simulink model "gm_uz_pmsm_model_vnl"  (R2023b)
settings: Solver=FixedStepAuto  StartTime=0.0  StopTime=0.05  RelTol=1e-3
PreLoadFcn:
  | uz_pmsm_model_init_parameter
PostLoadFcn:
  | % Import the data from Excel for a lookup table
  | FluxMapData = readtable('C:\Users\Philipp\ultrazohm\ultrazohm_sw\ip_cores\uz_pmsm_model\FluxMapData_2023-05-26_13-07-57.csv');
  | % Row indices for lookup table
  | d_current_in_d_axis = FluxMapData(8:27,1:end);
  | % Column indices for lookup table
  | q_current_in_d_axis = FluxMapData(29:48,1:end);
  | % Output values for lookup table
  | d_Flux_d_axis = FluxMapData(50:69,1:end);
undefined symbols (not defined in the file or in its folder): ad1, ad2, ad3, ad4, ad5, ad6, aq1, aq2, aq3, aq4, aq5, aq6, d_current_d_Flux, d_current_q_Flux, entkopplung_dynamic, entkopplung_linear, entkopplung_static, Fid1_Giq1, Fid2_Giq2, Flux_d, Flux_q, friction_coefficient, inertia, Ki_Bo_d, Ki_Bo_q, Kp_Bo_d, Kp_Bo_q, L_d, L_q, Ldq, parameter_nachfuerung, polepair, praediktion_entkopplung_nonlinear, psi_pm, q_current_d_Flux, q_current_q_Flux, R_1, simulate_mechanical, simulate_nonlinear_modell, simulate_open_loop, static_friction_torque, tau_sum, ts, ts_regler
libraries: hdlmdlgenlib x16, slpidlib x6, simulink x4
(part 2 of 5)

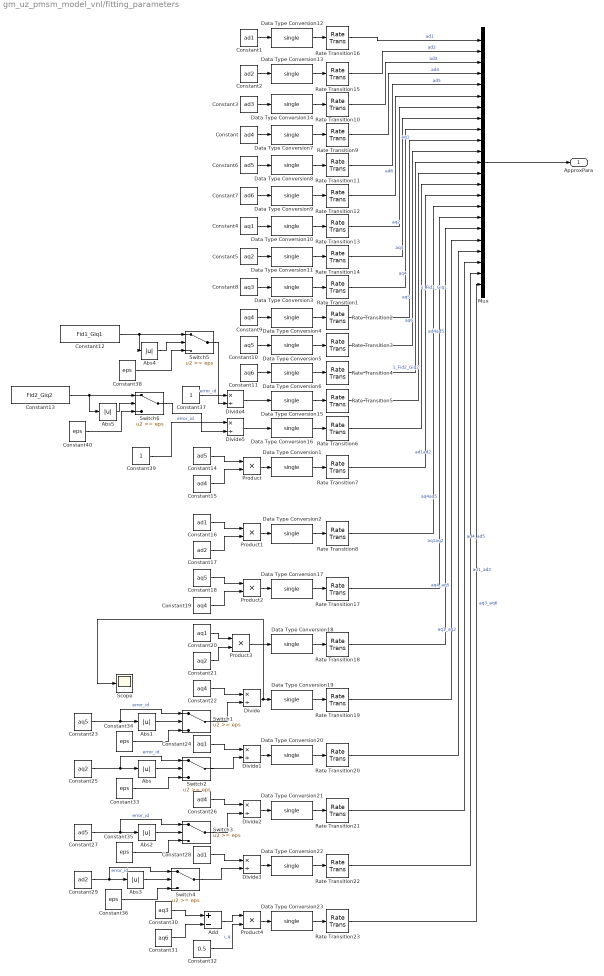
== system gm_uz_pmsm_model_vnl/fitting_parameters ==
  Abs{,1..5} (6 alike) : Abs  SaturateOnIntegerOverflow=off
  Add : Sum  Inputs=+-
  Constant : Constant  Value=ad4
  Constant1 : Constant  Value=ad1
  Constant10 : Constant  Value=aq5
  Constant11 : Constant  Value=aq6
  Constant12 : Constant  Value=Fid1_Giq1
  Constant13 : Constant  Value=Fid2_Giq2
  Constant14 : Constant  Value=ad5
  Constant15 : Constant  Value=ad4
  Constant16 : Constant  Value=ad1
  Constant17 : Constant  Value=ad2
  Constant18 : Constant  Value=aq5
  Constant19 : Constant  Value=aq4
  Constant2 : Constant  Value=ad2
  Constant20 : Constant  Value=aq1
  Constant21 : Constant  Value=aq2
  Constant22 : Constant  Value=aq4
  Constant23 : Constant  Value=aq5
  Constant24 : Constant  Value=aq1
  Constant25 : Constant  Value=aq2
  Constant26 : Constant  Value=ad4
  Constant27 : Constant  Value=ad5
  Constant28 : Constant  Value=ad1
  Constant29 : Constant  Value=ad2
  Constant3 : Constant  Value=ad3
  Constant30 : Constant  Value=aq3
  Constant31 : Constant  Value=aq6
  Constant32 : Constant  Value=0.5  OutDataTypeStr=double  SampleTime=-1
  Constant{33..36,38,40} (6 alike) : Constant  Value=eps  SampleTime=ts_regler
  Constant37 : Constant
  Constant39 : Constant
  Constant4 : Constant  Value=aq1
  Constant5 : Constant  Value=aq2
  Constant6 : Constant  Value=ad5
  Constant7 : Constant  Value=ad6
  Constant8 : Constant  Value=aq3
  Constant9 : Constant  Value=aq4
  Data Type Conversion{1..23} (23 alike) : DataTypeConversion  OutDataTypeStr=single  SaturateOnIntegerOverflow=off  RndMeth=Floor
  Divide{,1..5} (6 alike) : Product  Inputs=*/
  Mux : Mux  Inputs=23
  Product{,1..4} (5 alike) : Product
  Rate Transition{1..23} (23 alike) : RateTransition  OutPortSampleTime=ts
  Scope : Scope
  Switch{1..6} (6 alike) : Switch  Threshold=eps  SaturateOnIntegerOverflow=off  InputSameDT=off
  ApproxPara : Outport
  wires:
  Constant1/1 -> Data Type Conversion12/1
  Constant/1 -> Data Type Conversion7/1
  Rate Transition10/1 -> Mux/3  "ad3"
  Rate Transition14/1 -> Mux/8  "aq2"
  Constant3/1 -> Data Type Conversion14/1
  Rate Transition12/1 -> Mux/6  "ad6"
  Rate Transition16/1 -> Mux/1  "ad1"
  Rate Transition13/1 -> Mux/7  "aq1"
  Constant5/1 -> Data Type Conversion11/1
  Constant7/1 -> Data Type Conversion9/1
  Rate Transition15/1 -> Mux/2  "ad2"
  Rate Transition9/1 -> Mux/4  "ad4"
  Constant6/1 -> Data Type Conversion8/1
  Constant4/1 -> Data Type Conversion10/1
  Rate Transition11/1 -> Mux/5  "ad5"
  Constant2/1 -> Data Type Conversion13/1
  Rate Transition1/1 -> Mux/9  "aq3"
  Constant8/1 -> Data Type Conversion3/1
  Rate Transition2/1 -> Mux/10  "aq4"
  Constant9/1 -> Data Type Conversion4/1
  Rate Transition3/1 -> Mux/11  "aq5"
  Constant10/1 -> Data Type Conversion5/1
  Rate Transition4/1 -> Mux/12  "aq6"
  Constant11/1 -> Data Type Conversion6/1
  Rate Transition5/1 -> Mux/13  "1_Fid1_Giq1"
  Rate Transition6/1 -> Mux/14  "1_Fid2_Giq2"
  Data Type Conversion11/1 -> Rate Transition14/1
  Data Type Conversion10/1 -> Rate Transition13/1
  Data Type Conversion9/1 -> Rate Transition12/1
  Data Type Conversion12/1 -> Rate Transition16/1
  Data Type Conversion13/1 -> Rate Transition15/1
  Data Type Conversion14/1 -> Rate Transition10/1
  Data Type Conversion7/1 -> Rate Transition9/1
  Data Type Conversion8/1 -> Rate Transition11/1
  Data Type Conversion3/1 -> Rate Transition1/1
  Data Type Conversion4/1 -> Rate Transition2/1
  Data Type Conversion5/1 -> Rate Transition3/1
  Data Type Conversion6/1 -> Rate Transition4/1
  Data Type Conversion15/1 -> Rate Transition5/1
  Data Type Conversion16/1 -> Rate Transition6/1
  Constant14/1 -> Product/1
  Constant15/1 -> Product/2
  Product/1 -> Data Type Conversion1/1
  Data Type Conversion1/1 -> Rate Transition7/1
  Rate Transition7/1 -> Mux/15  "ad4ad5"
  Rate Transition8/1 -> Mux/16  "ad1ad2"
  Constant16/1 -> Product1/1
  Constant17/1 -> Product1/2
  Data Type Conversion2/1 -> Rate Transition8/1
  Product1/1 -> Data Type Conversion2/1
  Constant18/1 -> Product2/1
  Constant19/1 -> Product2/2
  Data Type Conversion17/1 -> Rate Transition17/1
  Product2/1 -> Data Type Conversion17/1
  Rate Transition18/1 -> Mux/18  "aq1aq2"
  Product3/1 -> Data Type Conversion18/1
  Data Type Conversion18/1 -> Rate Transition18/1
  Constant21/1 -> Product3/2
  Constant20/1 -> Product3/1
  Rate Transition17/1 -> Mux/17  "aq4aq5"
  Divide/1 -> Scope/1, Data Type Conversion19/1
  Data Type Conversion19/1 -> Rate Transition19/1
  Constant22/1 -> Divide/1
  Rate Transition19/1 -> Mux/19  "aq4_aq5"
  Constant24/1 -> Divide1/1
  Rate Transition20/1 -> Mux/20  "aq1_aq2"
  Divide1/1 -> Data Type Conversion20/1
  Data Type Conversion20/1 -> Rate Transition20/1
  Data Type Conversion21/1 -> Rate Transition21/1
  Divide2/1 -> Data Type Conversion21/1
  Rate Transition21/1 -> Mux/21  "ad4_ad5"
  Constant26/1 -> Divide2/1
  Constant28/1 -> Divide3/1
  Rate Transition22/1 -> Mux/22  "ad1_ad2"
  Divide3/1 -> Data Type Conversion22/1
  Data Type Conversion22/1 -> Rate Transition22/1
  Data Type Conversion23/1 -> Rate Transition23/1
  Constant30/1 -> Add/1
  Constant31/1 -> Add/2
  Rate Transition23/1 -> Mux/23  "aq3_aq6"
  Product4/1 -> Data Type Conversion23/1
  Constant32/1 -> Product4/2  "i_q"
  Add/1 -> Product4/1
  Mux/1 -> ApproxPara/1
  Constant25/1 -> Switch2/1, Abs/1  "error_id"
  Switch2/1 -> Divide1/2
  Abs/1 -> Switch2/2
  Constant33/1 -> Switch2/3
  Constant23/1 -> Switch1/1, Abs1/1  "error_id"
  Switch1/1 -> Divide/2
  Abs1/1 -> Switch1/2
  Constant34/1 -> Switch1/3
  Constant27/1 -> Switch3/1, Abs2/1  "error_id"
  Switch3/1 -> Divide2/2
  Abs2/1 -> Switch3/2
  Constant35/1 -> Switch3/3
  Constant29/1 -> Switch4/1, Abs3/1  "error_id"
  Switch4/1 -> Divide3/2
  Abs3/1 -> Switch4/2
  Constant36/1 -> Switch4/3
  Abs4/1 -> Switch5/2
  Constant38/1 -> Switch5/3
  Divide4/1 -> Data Type Conversion15/1
  Switch5/1 -> Divide4/2
  Constant12/1 -> Abs4/1, Switch5/1
  Constant37/1 -> Divide4/1  "error_id"
  Constant39/1 -> Divide5/1  "error_id"
  Constant13/1 -> Abs5/1, Switch6/1
  Constant40/1 -> Switch6/3
  Abs5/1 -> Switch6/2
  Divide5/1 -> Data Type Conversion16/1
  Switch6/1 -> Divide5/2

== system gm_uz_pmsm_model_vnl/model_parameters1 ==
  Bus Creator : BusCreator  Inputs=8
  Constant : Constant  Value=L_d
  Constant6 : Constant  Value=L_q
  Constant7 : Constant  Value=R_1
  Constant8 : Constant  Value=polepair
  Constant9 : Constant  Value=psi_pm
  Data Type Conversion{7..14} (8 alike) : DataTypeConversion  OutDataTypeStr=single  SaturateOnIntegerOverflow=off  RndMeth=Floor
  J : Constant  Value=1/inertia
  M_R0 : Constant  Value=static_friction_torque
  Rate Transition{9..16} (8 alike) : RateTransition  OutPortSampleTime=ts
  mu : Constant  Value=friction_coefficient
  Out1 : Outport
  wires:
  Data Type Conversion12/1 -> Rate Transition16/1
  Data Type Conversion7/1 -> Rate Transition9/1
  Rate Transition10/1 -> Bus Creator/3  "M_R0"
  Rate Transition14/1 -> Bus Creator/8  "psi_pm"
  Data Type Conversion14/1 -> Rate Transition10/1
  Rate Transition12/1 -> Bus Creator/6  "R_1"
  Rate Transition16/1 -> Bus Creator/1  "1_J"
  Rate Transition13/1 -> Bus Creator/7  "polepair"
  Bus Creator/1 -> Out1/1
  Data Type Conversion11/1 -> Rate Transition14/1
  Constant8/1 -> Data Type Conversion10/1
  Data Type Conversion9/1 -> Rate Transition12/1
  Rate Transition15/1 -> Bus Creator/2  "mu"
  Constant6/1 -> Data Type Conversion8/1
  Rate Transition9/1 -> Bus Creator/4  "1_L_d"
  J/1 -> Data Type Conversion12/1
  Data Type Conversion8/1 -> Rate Transition11/1
  Data Type Conversion10/1 -> Rate Transition13/1
  mu/1 -> Data Type Conversion13/1
  M_R0/1 -> Data Type Conversion14/1
  Rate Transition11/1 -> Bus Creator/5  "1_L_q"
  Data Type Conversion13/1 -> Rate Transition15/1
  Constant7/1 -> Data Type Conversion9/1
  Constant9/1 -> Data Type Conversion11/1
  Constant/1 -> Data Type Conversion7/1

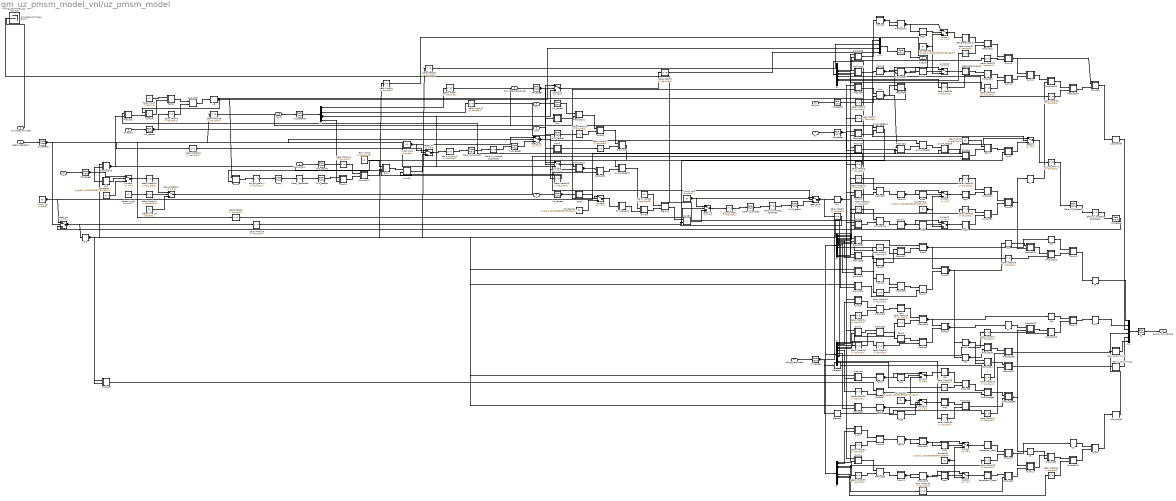
== system gm_uz_pmsm_model_vnl/uz_pmsm_model ==
  reset_integrators : Inport  OutDataTypeStr=boolean  PortDimensions=1  SampleTime=2e-06
  simulate_mechanical : Inport  Port=2  OutDataTypeStr=boolean  PortDimensions=1  SampleTime=2e-06
  simulate_nonlinear : Inport  Port=3  OutDataTypeStr=boolean  PortDimensions=1  SampleTime=2e-06
  reciprocal_J : Inport  Port=4  OutDataTypeStr=single  PortDimensions=1  SampleTime=2e-06
  mu : Inport  Port=5  OutDataTypeStr=single  PortDimensions=1  SampleTime=2e-06
  M_n0 : Inport  Port=6  OutDataTypeStr=single  PortDimensions=1  SampleTime=2e-06
  R1 : Inport  Port=7  OutDataTypeStr=single  PortDimensions=1  SampleTime=2e-06
  polepairs : Inport  Port=8  OutDataTypeStr=single  PortDimensions=1  SampleTime=2e-06
  Ld : Inport  Port=9  OutDataTypeStr=single  PortDimensions=1  SampleTime=2e-06
  Lq : Inport  Port=10  OutDataTypeStr=single  PortDimensions=1  SampleTime=2e-06
  psi_pm : Inport  Port=11  OutDataTypeStr=single  PortDimensions=1  SampleTime=2e-06
  fitting_parameter : Inport  Port=12  OutDataTypeStr=single  PortDimensions=[23]  SampleTime=2e-06
  inputs : Inport  Port=13  OutDataTypeStr=single  PortDimensions=[4]  SampleTime=2e-06
  Abs : Subsystem
      mask Display: disp('NFP\nabs');
  Constant{1..2,21..24} (6 alike) : Constant  Value=single(1.1920928955078125e-07)  OutDataTypeStr=single  SampleTime=1e-08
  Delay : RateTransition  OutPortSampleTimeOpt=Multiple of input port sample time  OutPortSampleTimeMultiple=200
  Delay1_lowered : RateTransition  OutPortSampleTimeOpt=Multiple of input port sample time  OutPortSampleTimeMultiple=200
  Delay1_lowered1 : RateTransition  OutPortSampleTimeOpt=Multiple of input port sample time  OutPortSampleTimeMultiple=200
  Delay1_lowered2 : RateTransition  OutPortSampleTimeOpt=Multiple of input port sample time  OutPortSampleTimeMultiple=200
  Delay1_lowered_absorbed : Delay  DelayLength=0
  Delay1_lowered_absorbed1 : Delay  DelayLength=0
  Delay1_lowered_absorbed2 : Delay  DelayLength=0
  Delay_absorbed : Delay  DelayLength=0
  Divide : Subsystem
      mask Display: disp('NFP\nmul');
  Divide1 : Subsystem
      mask Display: disp('NFP\nmul');
  Divide_recip : Subsystem
      mask Display: disp('NFP\nmath');
  Factor : Subsystem
      mask Display: disp('NFP\nmul');
  Factor_const : Constant  Value=single(1.5)  OutDataTypeStr=single  SampleTime=1e-08
  Gain : Subsystem
      mask Display: disp('NFP\nmul');
  Gain7 : Subsystem
      mask Display: disp('NFP\nmul');
  Gain71 : Subsystem
      mask Display: disp('NFP\nmul');
  Gain7_const : Constant  Value=single(2e-06)  OutDataTypeStr=single  SampleTime=1e-08
  Gain7_const1 : Constant  Value=single(2e-06)  OutDataTypeStr=single  SampleTime=1e-08
  Gain_const : Constant  Value=single(2e-06)  OutDataTypeStr=single  SampleTime=1e-08
  Gain_unaryminus : Subsystem
      mask Display: disp('NFP\numinus');
  Gain_unaryminus1 : Subsystem
      mask Display: disp('NFP\numinus');
  Initial_Val : Constant  Value=single(0)  OutDataTypeStr=single  SampleTime=1e-08
  Initial_Val1 : Constant  Value=single(0)  OutDataTypeStr=single  SampleTime=1e-08
  Initial_Val2 : Constant  Value=single(0)  OutDataTypeStr=single  SampleTime=1e-08
  Ldd_modell : hdlmdlgenlib/Buffer
  Log : Subsystem
      mask Display: disp('NFP\nmath');
  Log1 : Subsystem
      mask Display: disp('NFP\nmath');
  Log11 : Subsystem
      mask Display: disp('NFP\nmath');
  Log2 : Subsystem
      mask Display: disp('NFP\nmath');
  Lqq_modell : hdlmdlgenlib/Buffer
  Product : Subsystem
      mask Display: disp('NFP\nmul');
  Product1 : Subsystem
      mask Display: disp('NFP\nmul');
  Product10 : Subsystem
      mask Display: disp('NFP\nmul');
  Product101 : Subsystem
      mask Display: disp('NFP\nmul');
  Product102 : Subsystem
      mask Display: disp('NFP\nmul');
  Product103 : Subsystem
      mask Display: disp('NFP\nmul');
  Product104 : Subsystem
      mask Display: disp('NFP\nmul');
  Product11 : Subsystem
      mask Display: disp('NFP\nmul');
  Product110 : Subsystem
      mask Display: disp('NFP\nmul');
  Product111 : Subsystem
      mask Display: disp('NFP\nmul');
  Product12 : Subsystem
      mask Display: disp('NFP\nmul');
  Product121 : Subsystem
      mask Display: disp('NFP\nmul');
  Product13 : Subsystem
      mask Display: disp('NFP\nmul');
  Product131 : Subsystem
      mask Display: disp('NFP\nmul');
  Product14 : Subsystem
      mask Display: disp('NFP\nmul');
  Product141 : Subsystem
      mask Display: disp('NFP\nmul');
  Product15 : Subsystem
      mask Display: disp('NFP\nmul');
  Product151 : Subsystem
      mask Display: disp('NFP\nmul');
  Product16 : Subsystem
      mask Display: disp('NFP\nmul');
  Product17 : Subsystem
      mask Display: disp('NFP\nmul');
  Product18 : Subsystem
      mask Display: disp('NFP\nmul');
  Product19 : Subsystem
      mask Display: disp('NFP\nmul');
  Product2 : Subsystem
      mask Display: disp('NFP\nmul');
  Product20 : Subsystem
      mask Display: disp('NFP\nmul');
  Product201 : Subsystem
      mask Display: disp('NFP\nmul');
  Product202 : Subsystem
      mask Display: disp('NFP\nmul');
  Product203 : Subsystem
      mask Display: disp('NFP\nmul');
  Product204 : Subsystem
      mask Display: disp('NFP\nmul');
  Product205 : Subsystem
      mask Display: disp('NFP\nmul');
  Product206 : Subsystem
      mask Display: disp('NFP\nmul');
  Product207 : Subsystem
      mask Display: disp('NFP\nmul');
  Product21 : Subsystem
      mask Display: disp('NFP\nmul');
  Product22 : Subsystem
      mask Display: disp('NFP\nmul');
  Product23 : Subsystem
      mask Display: disp('NFP\nmul');
  Product24 : Subsystem
      mask Display: disp('NFP\nmul');
  Product25 : Subsystem
      mask Display: disp('NFP\nmul');
  Product3 : Subsystem
      mask Display: disp('NFP\nmul');
  Product31 : Subsystem
      mask Display: disp('NFP\nmul');
  Product32 : Subsystem
      mask Display: disp('NFP\nmul');
  Product33 : Subsystem
      mask Display: disp('NFP\nmul');
  Product34 : Subsystem
      mask Display: disp('NFP\nmul');
  Product35 : Subsystem
      mask Display: disp('NFP\nmul');
  Product4 : Subsystem
      mask Display: disp('NFP\nmul');
  Product41 : Subsystem
      mask Display: disp('NFP\nmul');
  Product42 : Subsystem
      mask Display: disp('NFP\nmul');
  Product43 : Subsystem
      mask Display: disp('NFP\nmul');
  Product5 : Subsystem
      mask Display: disp('NFP\nmul');
  Product51 : Subsystem
      mask Display: disp('NFP\nmul');
  Product52 : Subsystem
      mask Display: disp('NFP\nmul');
  Product6 : Subsystem
      mask Display: disp('NFP\nmul');
  Product61 : Subsystem
      mask Display: disp('NFP\nmul');
  Product7 : Subsystem
      mask Display: disp('NFP\nmul');
  Product71 : Subsystem
      mask Display: disp('NFP\nmul');
  Product8 : Subsystem
      mask Display: disp('NFP\nmul');
  Product9 : Subsystem
      mask Display: disp('NFP\nmul');
  Product91 : Subsystem
      mask Display: disp('NFP\nmul');
  Product92 : Subsystem
      mask Display: disp('NFP\nmul');
  Reciprocal1_recip : Subsystem
      mask Display: disp('NFP\nmath');
  Reciprocal1_recip1 : Subsystem
      mask Display: disp('NFP\nmath');
  Reciprocal_recip : Subsystem
      mask Display: disp('NFP\nmath');
  Reciprocal_recip1 : Subsystem
      mask Display: disp('NFP\nmath');
  Selector : Selector  IndexOptions=Index vector (dialog)  Indices=double(14)  OutputSizes=double(1)
  Selector1 : Selector  IndexOptions=Index vector (dialog)  Indices=double(13)  OutputSizes=double(1)
  Sign1 : Subsystem
      mask Display: disp('NFP\nsignum');
  Sum : Subsystem
      mask Display: disp('NFP\nadd');
  Sum1 : Subsystem
      mask Display: disp('NFP\nadd');
  Sum10 : Subsystem
      mask Display: disp('NFP\nadd');
  Sum101 : Subsystem
      mask Display: disp('NFP\nadd');
  Sum11 : Subsystem
      mask Display: disp('NFP\nadd');
  Sum12 : Subsystem
      mask Display: disp('NFP\nadd');
  Sum13 : Subsystem
      mask Display: disp('NFP\nadd');
  Sum14 : Subsystem
      mask Display: disp('NFP\nadd');
  Sum2 : Subsystem
      mask Display: disp('NFP\nadd');
  Sum21 : Subsystem
      mask Display: disp('NFP\nadd');
  Sum22 : Subsystem
      mask Display: disp('NFP\nadd');
  Sum23 : Subsystem
      mask Display: disp('NFP\nadd');
  Sum24 : Subsystem
      mask Display: disp('NFP\nadd');
  Sum3 : Subsystem
      mask Display: disp('NFP\nadd');
  Sum31 : Subsystem
      mask Display: disp('NFP\nadd');
  Sum32 : Subsystem
      mask Display: disp('NFP\nadd');
  Sum33 : Subsystem
      mask Display: disp('NFP\nadd');
  Sum3_stage2 : Subsystem
      mask Display: disp('NFP\nadd');
  Sum3_stage21 : Subsystem
      mask Display: disp('NFP\nadd');
  Sum3_stage3 : Subsystem
      mask Display: disp('NFP\nadd');
  Sum3_stage31 : Subsystem
      mask Display: disp('NFP\nadd');
  Sum4 : Subsystem
      mask Display: disp('NFP\nadd');
  Sum41 : Subsystem
      mask Display: disp('NFP\nadd');
  Sum4_stage2 : Subsystem
      mask Display: disp('NFP\nadd');
  Sum4_stage3 : Subsystem
      mask Display: disp('NFP\nadd');
  Sum5 : Subsystem
      mask Display: disp('NFP\nadd');
  Sum51 : Subsystem
      mask Display: disp('NFP\nadd');
  Sum52 : Subsystem
      mask Display: disp('NFP\nadd');
  Sum53 : Subsystem
      mask Display: disp('NFP\nadd');
  Sum6 : Subsystem
      mask Display: disp('NFP\nadd');
  Sum7 : Subsystem
      mask Display: disp('NFP\nadd');
  Sum71 : Subsystem
      mask Display: disp('NFP\nadd');
  Sum8 : Subsystem
      mask Display: disp('NFP\nadd');
  Switch{,1..6,8,11..14} (12 alike) : Switch  Criteria=u2 ~= 0  Threshold=double(0)  OutDataTypeStr=single  SampleTime=1e-08  SaturateOnIntegerOverflow=off  InputSameDT=off
  Tanh : Subsystem
      mask Display: disp('NFP\ntrig');
  Tanh1 : Subsystem
      mask Display: disp('NFP\ntrig');
  Tanh11 : Subsystem
      mask Display: disp('NFP\ntrig');
  Tanh12 : Subsystem
      mask Display: disp('NFP\ntrig');
  Tanh13 : Subsystem
      mask Display: disp('NFP\ntrig');
  Tanh2 : Subsystem
      mask Display: disp('NFP\ntrig');
  Tanh21 : Subsystem
      mask Display: disp('NFP\ntrig');
  Tanh3 : Subsystem
      mask Display: disp('NFP\ntrig');
  Tanh31 : Subsystem
      mask Display: disp('NFP\ntrig');
  Tanh4 : Subsystem
      mask Display: disp('NFP\ntrig');
  Tanh41 : Subsystem
      mask Display: disp('NFP\ntrig');
  Tanh5 : Subsystem
      mask Display: disp('NFP\ntrig');
  abs : Subsystem
      mask Display: disp('NFP\nabs');
  abs1 : Subsystem
      mask Display: disp('NFP\nabs');
  abs2 : Subsystem
      mask Display: disp('NFP\nabs');
  abs3 : Subsystem
      mask Display: disp('NFP\nabs');
  abs4 : Subsystem
      mask Display: disp('NFP\nabs');
  abs5 : Subsystem
      mask Display: disp('NFP\nabs');
  abs6 : Subsystem
      mask Display: disp('NFP\nabs');
  abs7 : Subsystem
      mask Display: disp('NFP\nabs');
  abs8 : Subsystem
      mask Display: disp('NFP\nabs');
  abs9 : Subsystem
      mask Display: disp('NFP\nabs');
  crp_out_delay{,1..3} (4 alike) : Delay  DelayLength=double(1)  InitialCondition=0  SampleTime=1e-08
  default_value : Constant  Value=double(1)  OutDataTypeStr=single  SampleTime=1e-08
  delayMatch{,1..13,15..46} (46 alike) : Delay  DelayLength=double(1)  InitialCondition=0  SampleTime=1e-08
  delayMatch14 : Delay  DelayLength=double(30)  InitialCondition=0  SampleTime=1e-08
  fitting_parameter_13_term13 : Terminator
  i_q : hdlmdlgenlib/Buffer
  in0_repeat : RateTransition  Integrity=off  Deterministic=off  OutPortSampleTimeOpt=Multiple of input port sample time  OutPortSampleTimeMultiple=1/200
  in10_repeat : RateTransition  Integrity=off  Deterministic=off  OutPortSampleTimeOpt=Multiple of input port sample time  OutPortSampleTimeMultiple=1/200
  in11_repeat : RateTransition  Integrity=off  Deterministic=off  OutPortSampleTimeOpt=Multiple of input port sample time  OutPortSampleTimeMultiple=1/200
  in12_repeat : RateTransition  Integrity=off  Deterministic=off  OutPortSampleTimeOpt=Multiple of input port sample time  OutPortSampleTimeMultiple=1/200
  in13_repeat : RateTransition  Integrity=off  Deterministic=off  OutPortSampleTimeOpt=Multiple of input port sample time  OutPortSampleTimeMultiple=1/200
  in14_repeat : RateTransition  Integrity=off  Deterministic=off  OutPortSampleTimeOpt=Multiple of input port sample time  OutPortSampleTimeMultiple=1/200
  in15_repeat : RateTransition  Integrity=off  Deterministic=off  OutPortSampleTimeOpt=Multiple of input port sample time  OutPortSampleTimeMultiple=1/200
  in1_repeat : RateTransition  Integrity=off  Deterministic=off  OutPortSampleTimeOpt=Multiple of input port sample time  OutPortSampleTimeMultiple=1/200
  in2_repeat : RateTransition  Integrity=off  Deterministic=off  OutPortSampleTimeOpt=Multiple of input port sample time  OutPortSampleTimeMultiple=1/200
  in3_repeat : RateTransition  Integrity=off  Deterministic=off  OutPortSampleTimeOpt=Multiple of input port sample time  OutPortSampleTimeMultiple=1/200
  in4_repeat : RateTransition  Integrity=off  Deterministic=off  OutPortSampleTimeOpt=Multiple of input port sample time  OutPortSampleTimeMultiple=1/200
  in5_repeat : RateTransition  Integrity=off  Deterministic=off  OutPortSampleTimeOpt=Multiple of input port sample time  OutPortSampleTimeMultiple=1/200
  in6_repeat : RateTransition  Integrity=off  Deterministic=off  OutPortSampleTimeOpt=Multiple of input port sample time  OutPortSampleTimeMultiple=1/200
  in7_repeat : RateTransition  Integrity=off  Deterministic=off  OutPortSampleTimeOpt=Multiple of input port sample time  OutPortSampleTimeMultiple=1/200
  in8_repeat : RateTransition  Integrity=off  Deterministic=off  OutPortSampleTimeOpt=Multiple of input port sample time  OutPortSampleTimeMultiple=1/200
  in9_repeat : RateTransition  Integrity=off  Deterministic=off  OutPortSampleTimeOpt=Multiple of input port sample time  OutPortSampleTimeMultiple=1/200
  mux : Mux  Inputs=6
  mux1 : Mux
  reset_in : Switch  Criteria=u2 ~= 0  Threshold=double(0)  OutDataTypeStr=single  SampleTime=1e-08  SaturateOnIntegerOverflow=off  InputSameDT=off
  reset_in1 : Switch  Criteria=u2 ~= 0  Threshold=double(0)  OutDataTypeStr=single  SampleTime=1e-08  SaturateOnIntegerOverflow=off  InputSameDT=off
  reset_in2 : Switch  Criteria=u2 ~= 0  Threshold=double(0)  OutDataTypeStr=single  SampleTime=1e-08  SaturateOnIntegerOverflow=off  InputSameDT=off
  reset_out : Switch  Criteria=u2 ~= 0  Threshold=double(0)  OutDataTypeStr=single  SampleTime=1e-08  SaturateOnIntegerOverflow=off  InputSameDT=off
  reset_out1 : Switch  Criteria=u2 ~= 0  Threshold=double(0)  OutDataTypeStr=single  SampleTime=1e-08  SaturateOnIntegerOverflow=off  InputSameDT=off
  reset_out2 : Switch  Criteria=u2 ~= 0  Threshold=double(0)  OutDataTypeStr=single  SampleTime=1e-08  SaturateOnIntegerOverflow=off  InputSameDT=off
  select_signal : Constant  Value=double(1)  OutDataTypeStr=boolean  SampleTime=1e-08
  simulate_nonlinear_term2 : Terminator
  t : RateTransition  OutPortSampleTimeOpt=Multiple of input port sample time  OutPortSampleTimeMultiple=200
  t1 : RateTransition  OutPortSampleTimeOpt=Multiple of input port sample time  OutPortSampleTimeMultiple=200
  t{7..19} (13 alike) : hdlmdlgenlib/Buffer
  t{2..5} (4 alike) : Demux  Outputs=23
  t6 : Demux
  zero_protection : Switch  Criteria=u2 ~= 0  Threshold=double(0)  OutDataTypeStr=single  SampleTime=1e-08  SaturateOnIntegerOverflow=off  InputSameDT=off
  outputs : Outport  SampleTime=2e-06
  approx_flux_testing : Outport  Port=2  SampleTime=2e-06
  wires:
  default_value/1 -> zero_protection/3
  zero_protection/1 -> Divide1/2(In2)
  reset_out1/1 -> Switch5/1, Switch14/1, Sign1/1(In1), Abs/1(In1), delayMatch45/1
  Selector1/1 -> delayMatch43/1
  Selector/1 -> delayMatch42/1
  delayMatch46/1 -> reset_in1/2
  reset_out/1 -> delayMatch15/1, t13/1
  select_signal/1 -> delayMatch14/1
  Switch8/1 -> delayMatch13/1
  Switch14/1 -> delayMatch9/1
  delayMatch7/1 -> mux1/1
  delayMatch8/1 -> mux1/2
  delayMatch16/1 -> reset_in/2
  reset_out2/1 -> delayMatch1/1, t14/1
  delayMatch14/1 -> zero_protection/2
  Gain/1(Out1) -> Sum32/1(In1)
  Sum3_stage31/1(Out1) -> Divide/1(In1)
  Sum3_stage21/1(Out1) -> Sum3_stage31/1(In1)
  Divide_recip/1(Out1) -> Divide/2(In2)
  abs9/1(Out1) -> Switch6/2
  Sum53/1(Out1) -> reset_in2/3
  Product43/1(Out1) -> Sum3_stage21/2(In2)
  Product35/1(Out1) -> Sum33/1(In1)
  Sum33/1(Out1) -> Factor/2(In2)
  Sum8/1(Out1) -> crp_out_delay1/1
  Product42/1(Out1) -> Sum8/2(In2)
  Sum52/1(Out1) -> Product42/1(In1)
  Product121/1(Out1) -> Sum52/1(In1)
  Abs/1(Out1) -> Product121/2(In2)
  Sum32/1(Out1) -> reset_in1/3
  Product111/1(Out1) -> Gain/2(In2)
  Sum14/1(Out1) -> Product111/2(In2)
  Sign1/1(Out1) -> delayMatch11/1
  Product131/1(Out1) -> Product21/2(In2), Product34/1(In1)
  Product110/1(Out1) -> Product2/2(In2), Product34/2(In2)
  Product25/1(Out1) -> Tanh13/1(In1)
  Tanh13/1(Out1) -> Product151/1(In1), Product151/2(In2)
  Product151/1(Out1) -> Switch13/1, abs8/1(In1)
  abs8/1(Out1) -> Switch13/2
  Reciprocal1_recip1/1(Out1) -> Product33/1(In1)
  Sum41/1(Out1) -> Sum24/2(In2)
  Sum24/1(Out1) -> Product206/1(In1)
  Product206/1(Out1) -> Product207/1(In1)
  Sum13/1(Out1) -> Sum101/1(In1), Sum24/1(In1)
  Reciprocal_recip1/1(Out1) -> Product19/1(In1)
  abs7/1(Out1) -> Switch4/2
  Product141/1(Out1) -> Switch4/1, abs7/1(In1)
  Tanh31/1(Out1) -> Product141/1(In1), Product141/2(In2)
  Product18/1(Out1) -> Tanh31/1(In1)
  Sum4/1(Out1) -> Sum23/1(In1), t19/1
  Sum23/1(Out1) -> t12/1, t15/1
  Product204/1(Out1) -> Product205/1(In1)
  Product41/1(Out1) -> Sum51/1(In1)
  Tanh12/1(Out1) -> Product32/1(In1)
  Product24/1(Out1) -> Tanh12/1(In1)
  Sum12/1(Out1) -> Sum23/2(In2)
  Product61/1(Out1) -> Sum12/2(In2)
  Product52/1(Out1) -> Sum4/1(In1)
  Product17/1(Out1) -> Sum4/2(In2)
  Tanh5/1(Out1) -> Product17/1(In1)
  Product16/1(Out1) -> Tanh5/1(In1)
  Tanh41/1(Out1) -> Switch3/1, abs6/1(In1)
  abs6/1(Out1) -> Switch3/2
  abs5/1(Out1) -> Switch12/2
  Tanh21/1(Out1) -> Switch12/1, abs5/1(In1)
  Log11/1(Out1) -> Product91/2(In2)
  Product91/1(Out1) -> Sum51/2(In2)
  Log2/1(Out1) -> Product41/2(In2)
  Product202/1(Out1) -> Product203/1(In1)
  Sum22/1(Out1) -> t11/1, t17/1
  Product102/1(Out1) -> Product103/1(In1)
  Product13/1(Out1) -> Sum22/1(In1), t18/1
  Tanh/1(Out1) -> Product13/1(In1)
  Product11/1(Out1) -> Tanh/1(In1)
  Sum3/1(Out1) -> Product11/1(In1)
  Product4/1(Out1) -> Tanh2/1(In1)
  Tanh2/1(Out1) -> Switch2/1, abs4/1(In1)
  abs4/1(Out1) -> Switch2/2
  Log/1(Out1) -> Product6/1(In1)
  Product6/1(Out1) -> Sum3_stage2/1(In1)
  Sum3_stage2/1(Out1) -> Sum3_stage3/1(In1)
  Product12/1(Out1) -> Sum3_stage3/2(In2)
  Log1/1(Out1) -> Product12/1(In1)
  abs3/1(Out1) -> Switch11/2
  Product51/1(Out1) -> Tanh3/1(In1)
  Product7/1(Out1) -> Sum3_stage2/2(In2)
  Product8/1(Out1) -> Product7/1(In1)
  Product10/1(Out1) -> Product101/1(In1)
  Product1/1(Out1) -> Sum21/1(In1), t16/1
  Reciprocal1_recip/1(Out1) -> Product31/1(In1)
  abs2/1(Out1) -> Switch1/2
  Product15/1(Out1) -> Switch1/1, abs2/1(In1)
  Tanh11/1(Out1) -> Product15/1(In1), Product15/2(In2)
  Product23/1(Out1) -> Tanh11/1(In1)
  Sum11/1(Out1) -> Product23/1(In1)
  Product/1(Out1) -> Tanh4/1(In1)
  Sum2/1(Out1) -> Product/1(In1)
  Tanh4/1(Out1) -> Product14/1(In1), Product14/2(In2)
  Product14/1(Out1) -> Switch/1, abs1/1(In1)
  abs1/1(Out1) -> Switch/2
  Reciprocal_recip/1(Out1) -> Product1/1(In1)
  Tanh1/1(Out1) -> Product3/1(In1)
  Product22/1(Out1) -> Tanh1/1(In1)
  Sum1/1(Out1) -> Product22/1(In1)
  Product201/1(Out1) -> Gain_unaryminus1/1(In1)
  Product20/1(Out1) -> Product201/1(In1)
  Product9/1(Out1) -> Sum4_stage3/2(In2)
  Sum4_stage3/1(Out1) -> Divide1/1(In1)
  Sum4_stage2/1(Out1) -> Sum4_stage3/1(In1)
  Sum/1(Out1) -> Product35/1(In1), Product21/1(In1)
  Product5/1(Out1) -> Sum/1(In1)
  abs/1(Out1) -> Switch8/2
  Sum5/1(Out1) -> reset_in/3
  Product2/1(Out1) -> Sum33/2(In2)
  Gain7_const1/1 -> Gain71/1(In1)
  Factor_const/1 -> Factor/1(In1)
  Gain_const/1 -> Gain/1(In1)
  Gain7_const/1 -> Gain7/1(In1)
  t6/2 -> delayMatch12/1
  t6/1 -> delayMatch/1
  t5/18 -> delayMatch32/1
  t5/17 -> delayMatch34/1
  t5/14 -> delayMatch36/1
  t5/12 -> delayMatch35/1
  t5/9 -> delayMatch33/1
  t4/22 -> delayMatch21/1
  t4/21 -> delayMatch22/1
  t4/14 -> delayMatch23/1
  t4/10 -> delayMatch18/1
  t4/7 -> delayMatch17/1
  t4/5 -> delayMatch20/1
  t4/2 -> delayMatch19/1
  t3/23 -> delayMatch29/1
  t3/20 -> delayMatch28/1
  t3/19 -> delayMatch30/1
  t3/14 -> fitting_parameter_13_term13/1
  t3/13 -> delayMatch31/1
  t3/5 -> delayMatch26/1
  t3/4 -> delayMatch27/1
  t3/2 -> delayMatch24/1
  t3/1 -> delayMatch25/1
  t2/16 -> delayMatch38/1
  t2/15 -> delayMatch40/1
  t2/13 -> delayMatch41/1
  t2/5 -> delayMatch39/1
  t2/2 -> delayMatch37/1
  delayMatch10/1 -> Sum52/2(In2)
  delayMatch44/1 -> Product111/1(In1)
  delayMatch6/1 -> Product92/2(In2)
  delayMatch3/1 -> Sum/2(In2)
  delayMatch2/1 -> reset_in2/2
  t6/4 -> Sum14/2(In2)
  t6/3 -> Switch5/3, Switch14/3
  delayMatch12/1 -> Sum4_stage2/1(In1)
  delayMatch/1 -> Sum3_stage21/1(In1)
  Divide/1(Out1) -> Gain71/2(In2)
  Switch6/1 -> Divide_recip/1(In1)
  Constant24/1 -> Switch6/3
  Gain71/1(Out1) -> Sum53/1(In1)
  reset_in2/1 -> crp_out_delay/1
  Initial_Val2/1 -> reset_in2/1, reset_out2/1
  delayMatch1/1 -> Sum53/2(In2)
  t14/1 -> delayMatch5/1, delayMatch7/1, Product5/1(In1), Sum1/1(In1), Sum2/1(In1), Sum11/1(In1), Sum3/1(In1), Sum6/1(In1), Sum31/1(In1), Product43/2(In2)
  delayMatch5/1 -> Product2/1(In1)
  delayMatch4/1 -> Product35/2(In2)
  Factor/1(Out1) -> Product92/1(In1)
  Product92/1(Out1) -> i_q/1
  i_q/1 -> mux1/3, Sum8/1(In1)
  delayMatch45/1 -> Sum32/2(In2)
  reset_in1/1 -> crp_out_delay3/1
  Initial_Val1/1 -> reset_in1/1, reset_out1/1
  delayMatch11/1 -> Product42/2(In2)
  delayMatch9/1 -> mux1/4
  Switch5/1 -> Product131/1(In1)
  Product34/1(Out1) -> Sum3_stage31/2(In2)
  t13/1 -> delayMatch4/1, delayMatch8/1, Product9/1(In1), Product8/1(In1), Product8/2(In2), Product51/1(In1), Product4/1(In1), Product16/1(In1), Product52/1(In1), Product61/1(In1), Product24/1(In1), Product18/1(In1), Product25/1(In1), Product110/1(In1)
  Switch13/1 -> Reciprocal1_recip1/1(In1)
  Product33/1(Out1) -> Sum41/1(In1)
  Product207/1(Out1) -> Sum101/2(In2)
  Sum101/1(Out1) -> Lqq_modell/1
  Product19/1(Out1) -> Sum13/1(In1)
  Switch4/1 -> Reciprocal_recip1/1(In1)
  Constant23/1 -> Switch4/3, Switch13/3
  delayMatch32/1 -> Product19/2(In2)
  delayMatch34/1 -> Product33/2(In2)
  delayMatch36/1 -> Product207/2(In2)
  delayMatch35/1 -> Sum41/2(In2)
  t5/11 -> Product25/2(In2)
  delayMatch33/1 -> Sum13/2(In2)
  t5/8 -> Product18/2(In2)
  Lqq_modell/1 -> mux/3
  t8/1 -> mux/1
  Sum10/1(Out1) -> t8/1
  t19/1 -> Sum10/1(In1)
  t15/1 -> Product204/1(In1)
  Product205/1(Out1) -> Sum10/2(In2)
  Sum51/1(Out1) -> Product204/2(In2), t7/1
  delayMatch21/1 -> Product41/1(In1)
  delayMatch22/1 -> Product91/1(In1)
  delayMatch23/1 -> Product205/2(In2)
  t4/12 -> Product61/2(In2)
  t4/11 -> Product24/2(In2)
  delayMatch18/1 -> Product32/2(In2)
  t4/9 -> Product52/2(In2)
  t4/8 -> Product16/2(In2)
  delayMatch17/1 -> Product17/2(In2)
  t4/6 -> Sum6/2(In2)
  delayMatch20/1 -> Product104/1(In1)
  t4/3 -> Sum31/2(In2)
  delayMatch19/1 -> Product71/1(In1)
  Product32/1(Out1) -> Sum12/1(In1)
  Product71/1(Out1) -> Tanh41/1(In1)
  Sum31/1(Out1) -> Product71/2(In2)
  Switch3/1 -> Log2/1(In1)
  Constant22/1 -> Switch12/3, Switch3/3
  Switch12/1 -> Log11/1(In1)
  Product104/1(Out1) -> Tanh21/1(In1)
  Sum6/1(Out1) -> Product104/2(In2)
  t7/1 -> Product206/2(In2)
  t12/1 -> Product20/2(In2), Product202/2(In2)
  Product203/1(Out1) -> Gain_unaryminus/1(In1)
  delayMatch43/1 -> Product203/2(In2)
  t11/1 -> Product20/1(In1), Product202/1(In1)
  t17/1 -> Product102/1(In1)
  Product103/1(Out1) -> Sum71/2(In2)
  Sum71/1(Out1) -> t10/1
  t18/1 -> Sum71/1(In1)
  delayMatch29/1 -> Product7/2(In2)
  delayMatch28/1 -> Product6/2(In2)
  delayMatch30/1 -> Product12/2(In2)
  delayMatch31/1 -> Product103/2(In2)
  t3/11 -> Product51/2(In2)
  t3/8 -> Product4/2(In2)
  t3/6 -> Sum1/2(In2)
  delayMatch26/1 -> Product22/2(In2)
  delayMatch27/1 -> Product3/2(In2)
  t3/3 -> Sum3/2(In2)
  delayMatch24/1 -> Product11/2(In2)
  delayMatch25/1 -> Product13/2(In2)
  Switch2/1 -> Log/1(In1)
  Sum3_stage3/1(Out1) -> Product102/2(In2), t9/1
  Switch11/1 -> Log1/1(In1)
  Constant21/1 -> Switch11/3, Switch2/3
  Tanh3/1(Out1) -> Switch11/1, abs3/1(In1)
  t9/1 -> Product10/2(In2)
  Product101/1(Out1) -> Sum7/2(In2)
  Sum7/1(Out1) -> Ldd_modell/1
  t16/1 -> Sum7/1(In1)
  Sum21/1(Out1) -> Product10/1(In1)
  Product31/1(Out1) -> Sum21/2(In2)
  Switch1/1 -> Reciprocal1_recip/1(In1)
  delayMatch38/1 -> Product1/2(In2)
  delayMatch40/1 -> Product31/2(In2)
  delayMatch41/1 -> Product101/2(In2)
  t2/6 -> Sum11/2(In2)
  delayMatch39/1 -> Product23/2(In2)
  t2/3 -> Sum2/2(In2)
  delayMatch37/1 -> Product/2(In2)
  Switch/1 -> Reciprocal_recip/1(In1)
  Constant2/1 -> Switch/3, Switch1/3
  Ldd_modell/1 -> mux/4
  Product3/1(Out1) -> Sum22/2(In2)
  t10/1 -> mux/2
  delayMatch42/1 -> Product201/2(In2)
  Gain_unaryminus1/1(Out1) -> mux/5
  Gain_unaryminus/1(Out1) -> mux/6
  Product21/1(Out1) -> Sum4_stage2/2(In2)
  Divide1/1(Out1) -> Gain7/2(In2)
  delayMatch13/1 -> zero_protection/1
  Constant1/1 -> Switch8/3
  Gain7/1(Out1) -> Sum5/1(In1)
  reset_in/1 -> crp_out_delay2/1
  Initial_Val/1 -> reset_in/1, reset_out/1
  delayMatch15/1 -> Sum5/2(In2)
  crp_out_delay3/1 -> Delay1_lowered1/1
  crp_out_delay2/1 -> Delay1_lowered2/1
  crp_out_delay1/1 -> Delay/1
  crp_out_delay/1 -> Delay1_lowered/1
  in2_repeat/1 -> reset_out/3
  Delay1_lowered_absorbed2/1 -> in2_repeat/1
  Delay1_lowered2/1 -> Delay1_lowered_absorbed2/1
  in11_repeat/1 -> Sum14/1(In1)
  Delay_absorbed/1 -> in11_repeat/1
  Delay/1 -> Delay_absorbed/1
  in12_repeat/1 -> reset_out1/3
  Delay1_lowered_absorbed1/1 -> in12_repeat/1
  Delay1_lowered1/1 -> Delay1_lowered_absorbed1/1
  in14_repeat/1 -> reset_out2/3
  Delay1_lowered_absorbed/1 -> in14_repeat/1
  Delay1_lowered/1 -> Delay1_lowered_absorbed/1
  mux/1 -> t1/1
  mux1/1 -> t/1
  in15_repeat/1 -> t6/1
  in13_repeat/1 -> delayMatch10/1
  in10_repeat/1 -> delayMatch44/1
  in9_repeat/1 -> Switch5/2, Switch14/2
  in8_repeat/1 -> Product131/2(In2), delayMatch6/1
  in7_repeat/1 -> Selector/1, t2/1, t3/1, Selector1/1, t4/1, t5/1
  in6_repeat/1 -> Product9/2(In2), Product43/1(In1)
  in5_repeat/1 -> delayMatch3/1
  in4_repeat/1 -> Switch6/1, Product5/2(In2), abs9/1(In1)
  in3_repeat/1 -> Switch8/1, abs/1(In1), Product110/2(In2)
  in1_repeat/1 -> reset_out/2, reset_out2/2, reset_out1/2, delayMatch2/1, delayMatch16/1, delayMatch46/1
  in0_repeat/1 -> Product121/1(In1)
  t1/1 -> approx_flux_testing/1
  t/1 -> outputs/1
  inputs/1 -> in15_repeat/1
  fitting_parameter/1 -> in7_repeat/1
  psi_pm/1 -> in5_repeat/1
  Lq/1 -> in3_repeat/1
  Ld/1 -> in4_repeat/1
  polepairs/1 -> in8_repeat/1
  R1/1 -> in6_repeat/1
  M_n0/1 -> in13_repeat/1
  mu/1 -> in0_repeat/1
  reciprocal_J/1 -> in10_repeat/1
  simulate_nonlinear/1 -> simulate_nonlinear_term2/1
  simulate_mechanical/1 -> in9_repeat/1
  reset_integrators/1 -> in1_repeat/1

== system gm_uz_pmsm_model_vnl/uz_pmsm_model_vnl ==
  reset_integrators : Inport
  simulate_mechanical : Inport  Port=2
  simulate_nonlinear : Inport  Port=3
  reciprocal_J : Inport  Port=4
  mu : Inport  Port=5
  M_n0 : Inport  Port=6
  R1 : Inport  Port=7
  polepairs : Inport  Port=8
  Ld : Inport  Port=9
  Lq : Inport  Port=10
  psi_pm : Inport  Port=11
  fitting_parameter : Inport  Port=12
  inputs : Inport  Port=13
  Demux : Demux
  Mux : Mux
  Scope : Scope  NumInputPorts=2
  Switch : Switch  Criteria=u2 ~= 0  SaturateOnIntegerOverflow=off  InputSameDT=off
  Switch1 : Switch  Criteria=u2 ~= 0  SaturateOnIntegerOverflow=off  InputSameDT=off
  mechanical_system : Subsystem
  pmsm : Subsystem
  torque_calculation : Subsystem
  outputs : Outport
  approx_flux_testing : Outport  Port=2
  wires:
  pmsm/5(approx_flux_testing) -> approx_flux_testing/1
  fitting_parameter/1 -> pmsm/10(fitting_parameters)
  reciprocal_J/1 -> mechanical_system/5(reciprocal_J)
  M_n0/1 -> mechanical_system/4(M_n0)
  mu/1 -> mechanical_system/3(mu)
  psi_pm/1 -> pmsm/9(psi_pm)
  Lq/1 -> pmsm/8(Lq)
  Ld/1 -> pmsm/7(Ld)
  polepairs/1 -> pmsm/6(polepairs1), torque_calculation/4(polepairs)
  R1/1 -> pmsm/5(R2)
  simulate_nonlinear/1 -> pmsm/2(simulate_nonlinear)
  Mux/1 -> outputs/1
  inputs/1 -> Demux/1
  torque_calculation/1(M_Mi) -> Mux/3, mechanical_system/2(M_Mi)  "i_q"
  Switch1/1 -> Mux/4  "i_q"
  pmsm/1(I_d1) -> Scope/1, torque_calculation/1(I_d), Mux/1  "i_d"
  pmsm/4(I_q1) -> Scope/2, Mux/2, torque_calculation/5(I_q)  "i_q"
  mechanical_system/1(omega_mech) -> Switch1/1, Switch/1
  Demux/2 -> pmsm/4(u_q1)  "u_q"
  simulate_mechanical/1 -> Switch/2, Switch1/2
  Demux/1 -> pmsm/3(u_d1)  "u_d"
  pmsm/3(psi_q1) -> torque_calculation/3(psi_q)
  Demux/4 -> mechanical_system/6(load_torque)  "load_torque"
  pmsm/2(psi_d1) -> torque_calculation/2(psi_d)
  Switch/1 -> pmsm/11(omega_mech1)
  Demux/3 -> Switch/3, Switch1/3  "omega_mech"
  reset_integrators/1 -> mechanical_system/1(reset), pmsm/1(reset1)

== system gm_uz_pmsm_model_vnl/Compare/Assert_approx_flux_testing ==
  cosim : Inport
  dut : Inport  Port=2
  AssertEq : Assertion  StopWhenAssertionFail=off
  Compare To Zero : simulink/Logic and Bit Operations/Compare To Zero  relop===  OutDataTypeStr=boolean
  Constant1 : Constant  Value=0  OutDataTypeStr=Inherit: Inherit via back propagation  SampleTime=-1
  Counter : simulink/Sources/Counter Free-Running  NumBits=32  tsamp=-1
  IgnoreCycles : Constant  Value=2  OutDataTypeStr=Inherit: Inherit via back propagation  SampleTime=-1
  RelErrCheck : Subsystem
  Relational Operator : RelationalOperator  Operator=<  OutDataTypeStr=boolean  InputSameDT=off
  Switch : Switch  Criteria=u2 ~= 0  SaturateOnIntegerOverflow=off  InputSameDT=off
  Switch1 : Switch  Criteria=u2 ~= 0  SaturateOnIntegerOverflow=off  InputSameDT=off
  compare: approx_flux_testing : Scope  NumInputPorts=3
  wires:
  IgnoreCycles/1 -> Relational Operator/2
  Counter/1 -> Relational Operator/1
  dut/1 -> Switch/3  "dut ref"
  cosim/1 -> Switch1/3  "cosim"
  Relational Operator/1 -> Switch1/2, Switch/2
  Constant1/1 -> Switch1/1, Switch/1
  Switch/1 -> compare: approx_flux_testing/2, RelErrCheck/2(In2)
  Switch1/1 -> compare: approx_flux_testing/1, RelErrCheck/1(In1)
  RelErrCheck/1(Out1) -> AssertEq/1, Compare To Zero/1  "err"
  Compare To Zero/1 -> compare: approx_flux_testing/3

== system gm_uz_pmsm_model_vnl/Compare/Assert_outputs ==
  cosim : Inport
  dut : Inport  Port=2
  AssertEq : Assertion  StopWhenAssertionFail=off
  Compare To Zero : simulink/Logic and Bit Operations/Compare To Zero  relop===  OutDataTypeStr=boolean
  Constant1 : Constant  Value=0  OutDataTypeStr=Inherit: Inherit via back propagation  SampleTime=-1
  Counter : simulink/Sources/Counter Free-Running  NumBits=32  tsamp=-1
  IgnoreCycles : Constant  Value=2  OutDataTypeStr=Inherit: Inherit via back propagation  SampleTime=-1
  RelErrCheck : Subsystem
  Relational Operator : RelationalOperator  Operator=<  OutDataTypeStr=boolean  InputSameDT=off
  Switch : Switch  Criteria=u2 ~= 0  SaturateOnIntegerOverflow=off  InputSameDT=off
  Switch1 : Switch  Criteria=u2 ~= 0  SaturateOnIntegerOverflow=off  InputSameDT=off
  compare: outputs : Scope  NumInputPorts=3
  wires:
  IgnoreCycles/1 -> Relational Operator/2
  Counter/1 -> Relational Operator/1
  dut/1 -> Switch/3  "dut ref"
  cosim/1 -> Switch1/3  "cosim"
  Relational Operator/1 -> Switch1/2, Switch/2
  Constant1/1 -> Switch1/1, Switch/1
  Switch/1 -> compare: outputs/2, RelErrCheck/2(In2)
  Switch1/1 -> compare: outputs/1, RelErrCheck/1(In1)
  RelErrCheck/1(Out1) -> AssertEq/1, Compare To Zero/1  "err"
  Compare To Zero/1 -> compare: outputs/3

== system gm_uz_pmsm_model_vnl/Compare/CleanupScopes ==

== system gm_uz_pmsm_model_vnl/Compare/Enable ==

== system gm_uz_pmsm_model_vnl/Curren t_Controller_With_FluxMaps_OLD/Entkopplung_flags ==
  u_d_static : Inport
  u_q_static : Inport  Port=2
  u_d_praed : Inport  Port=3
  u_q_praed : Inport  Port=4
  u_d_lin : Inport  Port=5
  u_q_lin : Inport  Port=6
  u_d_dyn : Inport  Port=7
  u_q_dyn : Inport  Port=8
  0 : Constant  Value=0
  Switch{1..8} (8 alike) : Switch  Criteria=u2 > Threshold  SaturateOnIntegerOverflow=off  InputSameDT=off
  entkopplung_dynamic : Constant  Value=entkopplung_dynamic
  entkopplung_linear : Constant  Value=entkopplung_linear
  entkopplung_preadiktion : Constant  Value=praediktion_entkopplung_nonlinear
  entkopplung_static : Constant  Value=entkopplung_static
  u_d_entk : Outport
  u_q_entk : Outport  Port=2
  wires:
  Switch3/1 -> u_d_entk/1
  Switch4/1 -> Switch2/3
  entkopplung_preadiktion/1 -> Switch2/2, Switch3/2
  Switch1/1 -> Switch3/3
  u_d_praed/1 -> Switch3/1
  Switch2/1 -> u_q_entk/1
  u_q_praed/1 -> Switch2/1
  entkopplung_static/1 -> Switch4/2, Switch1/2
  u_d_static/1 -> Switch1/1
  u_d_lin/1 -> Switch5/1
  Switch5/1 -> Switch1/3
  entkopplung_linear/1 -> Switch6/2, Switch5/2
  entkopplung_dynamic/1 -> Switch8/2, Switch7/2
  0/1 -> Switch8/3, Switch7/3
  Switch6/1 -> Switch4/3
  u_q_static/1 -> Switch4/1
  u_q_lin/1 -> Switch6/1
  u_d_dyn/1 -> Switch7/1
  Switch8/1 -> Switch6/3
  u_q_dyn/1 -> Switch8/1
  Switch7/1 -> Switch5/3

== system gm_uz_pmsm_model_vnl/Curren t_Controller_With_FluxMaps_OLD/Entkopplungen ==
  u_q : Inport
  u_d : Inport  Port=2
  uq : Inport  Port=3
  ud : Inport  Port=4
  i_d : Inport  Port=5
  psi_d_LUT : Inport  Port=6
  psi_q_LUT : Inport  Port=7
  Ldq_LUT : Inport  Port=8
  Lqd_LUT : Inport  Port=9
  i_q : Inport  Port=10
  omega_m : Inport  Port=11
  Lineare_Entkopplung : Subsystem
  decoupling_praediktion : Subsystem
  dynamic_nonlinear_entkopplung1 : Subsystem
  static_nonlinear_entkopplung : Subsystem
  u_d_static : Outport
  u_q_static : Outport  Port=2
  u_d_prae : Outport  Port=3
  u_q_prae : Outport  Port=4
  u_d_lin : Outport  Port=5
  u_q_lin : Outport  Port=6
  u_d_dyn : Outport  Port=7
  u_q_dyn1 : Outport  Port=8
  wires:
  psi_d_LUT/1 -> static_nonlinear_entkopplung/1(psi_d), dynamic_nonlinear_entkopplung1/3(psi_d), decoupling_praediktion/9(psi_d)
  omega_m/1 -> dynamic_nonlinear_entkopplung1/7(omega_m), Lineare_Entkopplung/3(omega_m), static_nonlinear_entkopplung/3(omega_m), decoupling_praediktion/5(omega_m)
  psi_q_LUT/1 -> dynamic_nonlinear_entkopplung1/4(psi_q), decoupling_praediktion/8(psi_q), static_nonlinear_entkopplung/2(psi_q)
  u_q/1 -> decoupling_praediktion/4(u_q_1)
  i_d/1 -> dynamic_nonlinear_entkopplung1/1(i_d), Lineare_Entkopplung/1(i_d), decoupling_praediktion/1(i_d)
  i_q/1 -> dynamic_nonlinear_entkopplung1/2(i_q), Lineare_Entkopplung/2(i_q), decoupling_praediktion/3(i_q)
  ud/1 -> decoupling_praediktion/6(u_d_k)
  uq/1 -> decoupling_praediktion/7(u_q_k)
  u_d/1 -> decoupling_praediktion/2(u_d_1)
  static_nonlinear_entkopplung/1(u_d) -> u_d_static/1
  Lineare_Entkopplung/1(u_d) -> u_d_lin/1
  static_nonlinear_entkopplung/2(u_q) -> u_q_static/1
  decoupling_praediktion/1(u_d_entk) -> u_d_prae/1
  Lineare_Entkopplung/2(u_q) -> u_q_lin/1
  decoupling_praediktion/2(u_q_entk) -> u_q_prae/1
  dynamic_nonlinear_entkopplung1/1(u_d) -> u_d_dyn/1
  dynamic_nonlinear_entkopplung1/2(u_q) -> u_q_dyn1/1
  Ldq_LUT/1 -> dynamic_nonlinear_entkopplung1/5(Ldq_LUT)
  Lqd_LUT/1 -> dynamic_nonlinear_entkopplung1/6(Lqd_LUT)

== system gm_uz_pmsm_model_vnl/Curren t_Controller_With_FluxMaps_OLD/Psi_d_q ==
  I_d_set : Inport
  I_d : Inport  Port=2
  I_q_set : Inport  Port=3
  I_q : Inport  Port=4
  ApproxPara : Inport  Port=5
  Constant4 : Constant  Value="eps(\"single\")"  SampleTime=ts_regler
  Constant5 : Constant  Value="eps(\"single\")"  SampleTime=ts_regler
  Divide : Product  Inputs=*/
  Divide1 : Product  Inputs=*/
  Sum{1..2,4..5} (4 alike) : Sum  Inputs=|+-
  Switch2 : Switch  Criteria=u2 ~= 0  Threshold=eps  SaturateOnIntegerOverflow=off  InputSameDT=off
  Switch3 : Switch  Criteria=u2 ~= 0  Threshold=eps  SaturateOnIntegerOverflow=off  InputSameDT=off
  psid_approx : Subsystem
  psid_approx1 : Subsystem
  psiq_approx : Subsystem
  psiq_approx1 : Subsystem
  Ldd_approx : Outport
  Lqq_approx : Outport  Port=2
  psid : Outport  Port=3
  psi_q : Outport  Port=4
  wires:
  I_q/1 -> Sum1/2, psiq_approx1/2(Iq), psid_approx1/2(Iq), psid_approx/2(Iq)
  psid_approx/1(psid) -> Sum4/1  "psi_d_set"
  psiq_approx/1(psiq) -> Sum5/1  "psi_q_set"
  ApproxPara/1 -> psid_approx1/3(FittingParameters), psid_approx/3(FittingParameters), psiq_approx/3(FittingParameters), psiq_approx1/3(FittingParameters)
  I_d/1 -> psid_approx1/1(Id), psiq_approx1/1(Id), Sum2/2, psiq_approx/1(Id)
  psiq_approx1/1(psiq) -> psi_q/1, Sum5/2  "psi_q"
  psid_approx1/1(psid) -> psid/1, Sum4/2  "psi_d"
  Constant5/1 -> Switch3/3
  Switch2/1 -> Divide/2
  Switch3/1 -> Divide1/2
  Divide/1 -> Ldd_approx/1  "Ldd_approx"
  Divide1/1 -> Lqq_approx/1  "Lqq_approx"
  Constant4/1 -> Switch2/3
  Sum5/1 -> Divide1/1
  Sum4/1 -> Divide/1
  Sum2/1 -> Switch2/2, Switch2/1
  I_q_set/1 -> Sum1/1, psiq_approx/2(Iq)
  I_d_set/1 -> Sum2/1, psid_approx/1(Id)
  Sum1/1 -> Switch3/2, Switch3/1

== system gm_uz_pmsm_model_vnl/Curren t_Controller_With_FluxMaps_OLD/Psi_d_q1 ==
  I_d : Inport
  I_q : Inport  Port=2
  ApproxPara : Inport  Port=3
  Ldd_approx1 : Subsystem
  Lqq_approx1 : Subsystem
  psid_approx : Subsystem
  psiq_approx : Subsystem
  psi_d : Outport
  Ldd : Outport  Port=2
  psi_q : Outport  Port=3
  Lqq : Outport  Port=4
  wires:
  psid_approx/1(psid) -> psi_d/1  "psi_d"
  psiq_approx/1(psiq) -> psi_q/1  "psi_q"
  I_q/1 -> psid_approx/2(Iq), Lqq_approx1/2(Iq), psiq_approx/2(Iq)
  psid_approx/2(psiq_cross_s1_integrated) -> Ldd_approx1/1(psiq_cross_s1_integrated)
  I_d/1 -> Ldd_approx1/2(Id), psid_approx/1(Id), psiq_approx/1(Id)
  psiq_approx/2(psid_cross_s1_integrated) -> Lqq_approx1/1(psid_cross_s1_integrated)
  Ldd_approx1/1(Ldd) -> Ldd/1  "Ldd"
  Lqq_approx1/1(Lqq) -> Lqq/1  "Lqq"
  ApproxPara/1 -> psiq_approx/3(FittingParameters), Ldd_approx1/3(FittingParameters), psid_approx/3(FittingParameters), Lqq_approx1/3(FittingParameters)

== system gm_uz_pmsm_model_vnl/Curren t_Controller_With_FluxMaps_OLD/Psi_d_q2 ==
  I_d_set : Inport
  I_d : Inport  Port=2
  I_q_set : Inport  Port=3
  I_q : Inport  Port=4
  ApproxPara : Inport  Port=5
  Ldd_approx1 : Subsystem
  Lqq_approx1 : Subsystem
  Scope : Scope  NumInputPorts=3
  psid_approx : Subsystem
  psid_approx1 : Subsystem
  psiq_approx : Subsystem
  psiq_approx1 : Subsystem
  psi_d_set : Outport
  psi_q_set : Outport  Port=2
  psi_d_LUT : Outport  Port=3
  psi_q_LUT : Outport  Port=4
  Lqq : Outport  Port=5
  Ldd : Outport  Port=6
  wires:
  I_q/1 -> Lqq_approx1/2(Iq), psiq_approx1/2(Iq), psid_approx1/2(Iq), psid_approx/2(Iq)
  psid_approx/1(psid) -> psi_d_set/1  "psi_d"
  psiq_approx/1(psiq) -> psi_q_set/1  "psi_q"
  ApproxPara/1 -> Ldd_approx1/3(FittingParameters), Lqq_approx1/3(FittingParameters), psiq_approx1/3(FittingParameters), psid_approx/3(FittingParameters), psid_approx1/3(FittingParameters), psiq_approx/3(FittingParameters)
  I_q_set/1 -> psiq_approx/2(Iq)
  I_d_set/1 -> psid_approx/1(Id)
  I_d/1 -> psiq_approx/1(Id), Ldd_approx1/2(Id), psiq_approx1/1(Id), psid_approx1/1(Id)
  psiq_approx1/1(psiq) -> Scope/1, psi_q_LUT/1  "psi_q_test"
  psid_approx1/1(psid) -> psi_d_LUT/1  "psi_d"
  Ldd_approx1/1(Ldd) -> Ldd/1  "Ldd_test"
  Lqq_approx1/1(Lqq) -> Scope/3, Lqq/1  "Lqq_test"
  psiq_approx1/2(psid_cross_s1_integrated) -> Lqq_approx1/1(psid_cross_s1_integrated), Scope/2  "psid_cross_rück_test"
  psid_approx1/2(psiq_cross_s1_integrated) -> Ldd_approx1/1(psiq_cross_s1_integrated)

== system gm_uz_pmsm_model_vnl/Curren t_Controller_With_FluxMaps_OLD/Reglernachführung ==
  Flag : Inport
  deadtime : Inport  Port=2
  R_s : Inport  Port=3
  Ld : Inport  Port=4
  Lq : Inport  Port=5
  Ldd : Inport  Port=6
  Lqq : Inport  Port=7
  Product : Product
  Product1 : Product
  Product2 : Product
  Switch : Switch  Criteria=u2 > Threshold  SaturateOnIntegerOverflow=off  InputSameDT=off
  Switch1 : Switch  Criteria=u2 > Threshold  SaturateOnIntegerOverflow=off  InputSameDT=off
  K_p_d : Outport
  K_p_q : Outport  Port=2
  K_I : Outport  Port=3
  wires:
  Product/1 -> K_p_d/1
  Product1/1 -> K_p_q/1
  Product2/1 -> K_I/1
  deadtime/1 -> Product2/1, Product1/1, Product/2  "id_regler"
  R_s/1 -> Product2/2  "id_regler"
  Flag/1 -> Switch/2, Switch1/2
  Ld/1 -> Switch/3
  Switch/1 -> Product/1
  Lq/1 -> Switch1/3
  Switch1/1 -> Product1/2
  Ldd/1 -> Switch/1
  Lqq/1 -> Switch1/1
